simulink model "calculator"  (R2021a)
settings: Solver=FixedStepAuto  StartTime=0.0  StopTime=10.0  RelTol=1e-3
settings Model: Creator=user  LastModifiedBy=user
settings OptimizationCC: DefaultParameterBehavior=Inlined  EnhancedBackFolding=on  PassReuseOutputArgsAs=Individual arguments  ZeroExternalMemoryAtStartup=off  ZeroInternalMemoryAtStartup=off  OptimizeBlockOrder=speed  DifferentSizesBufferReuse=on  OptimizationCustomize=off  EfficientTunableParamExpr=on
settings DebuggingCC: ParameterTunabilityLossMsg=error
settings SFSimCC: MATLABDynamicMemAlloc=off
settings RTWCC: SystemTargetFile=ert.tlc  GenCodeOnly=on  TemplateMakefile=ert_default_tmf  GenerateReport=on  IncludeHyperlinkInReport=on  LaunchReport=on  GenerateTraceInfo=on
settings CodeAppCC: ForceParamTrailComments=on  IgnoreCustomStorageClasses=off  OperatorAnnotations=on  SimulinkDataObjDesc=on  SFDataObjDesc=on  InsertBlockDesc=on
settings ERTTargetCC: TargetLangStandard=C99 (ISO)  GenerateSampleERTMain=on  InlinedParameterPlacement=NonHierarchical  ERTCustomFileTemplate=example_file_process.tlc

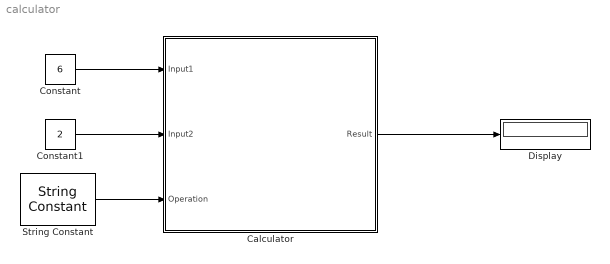
== system calculator ==
  Calculator : Stateflow chart  TreatAsAtomicUnit=on
  Constant : Constant  Value=6  OutDataTypeStr=uint16
  Constant1 : Constant  Value=2  OutDataTypeStr=uint16
  Display : Display
  String Constant : StringConstant  String='/'
  wires:
  Constant1/1 -> Calculator/2(Input2)
  String Constant/1 -> Calculator/3(Operation)
  Constant/1 -> Calculator/1(Input1)
  Calculator/1(Result) -> Display/1

== stateflow chart calculator/Calculator ==
  state Calculator(Input1,Input2) [function]
    (default) -> (junction 165) : % Switch
    (junction 165) -> (junction 169) [order 1] : [Operation == '+']
    (junction 165) -> (junction 168) [order 2]
    (junction 169) -> (junction 173) : {Result=Input1 + Input2 ;}
    (junction 173) -> (junction 188)
    (junction 188) -> (junction 192)
    (junction 168) -> (junction 167) [order 1] : [Operation == '-']
    (junction 168) -> (junction 172) [order 2]
    (junction 167) -> (junction 170) : {Result=Input1 - Input2;}
    (junction 170) -> (junction 192)
    (junction 192) -> (junction 193)
    (junction 172) -> (junction 179) [order 1] : [Operation == '*']
    (junction 172) -> (junction 176) [order 2]
    (junction 179) -> (junction 175) : {Result=Input1 * Input2 ;}
    (junction 175) -> (junction 193)
    (junction 193) -> (junction 194)
    (junction 176) -> (junction 178) [order 1] : [Operation == '/']
    (junction 176) -> (junction 177) [order 2]
    (junction 178) -> (junction 195)
    (junction 195) -> (junction 194) : {Result=Input1 / Input2 ;}
    (junction 194) -> (junction 190)
    (junction 190) -> (junction 177)
    (junction 177) -> (junction 207)
  (default) -> (junction 184) : {Calculator(Input1,Input2);}
  data: Input1 function_input double; Input2 function_input double; Input1 input uint16; Input2 input uint16; Result output uint16; Operation input
